simulink model "boostObserver_old"  (R2020a)
settings: Solver=VariableStepAuto  StartTime=0.0  StopTime=3.2  FixedStep=0.0005  MaxStep=9e-06  RelTol=1e-03  EnableMultiTasking=on
InitFcn:
  | kp=0.01;
  | ki=0.01;
  | 
  | k=2;
  | em=100000000;
  | GE=1/em;
  | GU=k*ki/GE;
  | GCE=k*kp/GU;
model workspace (MAT data in the model file):
  time = 0.8
values from neighbouring files (symbols this model uses):
  A1 = obj.boostConverter.A1    [BoostController.m]    (also in BoostConverter.m = [-obj.R/obj.L 0;0 -1/(obj.Ro*obj.C)]; BuckBoostConverter.m = [-obj.R/obj.L 0;0 -1/(obj.Ro*obj.C)]; obsmc.m = Asigma{1,1}; workspace_atual.mat = [-16.4  0; 0  -3.50877192982])
  A2 = obj.boostConverter.A2    [BoostController.m]    (also in BoostConverter.m = [-obj.R/obj.L -1/obj.L;1/obj.C -1/(obj.Ro*obj.C)]; BuckBoostConverter.m = [-obj.R/obj.L 1/obj.L;-1/obj.C -1/(obj.Ro*obj.C)]; obsmc.m = Asigma{1,2}; workspace_atual.mat = [-16.4  -200; 350.877192982  -3.50877192982])
  AlarmDeadTime = 0.50    (= 0.5)    [BoostFaultSimulation.m]    (also in workspace_atual.mat; workspace_certo.mat)
  B1 = obj.boostConverter.B1    [BoostController.m]    (also in BoostConverter.m = [1/obj.L;0]; BuckBoostConverter.m = [1/obj.L;0]; obsmc.m = Bsigma{1,1}; workspace_atual.mat = [200 0])
  boost_parameters = [obj.Ro,obj.R,obj.L,obj.C,obj.u]'    [BoostConverter.m]    (also in BuckBoostConverter.m; boostResults2Latex.m = boost.parameters(); workspace_atual.mat = [100 0.082 0.005 0.00285 190]; workspace_certo.mat = [100 0.082 0.005 0.00285 190])
  C = 1e-3    (= 0.001)    [boostResults2Latex.m]
  CiL = [0 1]    [workspace_atual.mat]    (also in workspace_certo.mat)
  Cmatrix = [1  0; 0  1]    [workspace_atual.mat]    (also in workspace_certo.mat)
  CVc = [1 0]    [workspace_atual.mat]    (also in workspace_certo.mat)
  D1 = [1  0; 0  1]    [workspace_atual.mat]    (also in workspace_certo.mat)
  FaultClass = 0    [BoostFaultSimulation.m]    (also in workspace_atual.mat = 1; workspace_certo.mat = 1)
  iLFaultSwitch = 0    [BoostFaultSimulation.m]    (also in workspace_atual.mat; workspace_certo.mat)
  iLFaultTime = 1.70    (= 1.7)    [BoostFaultSimulation.m]    (also in workspace_atual.mat; workspace_certo.mat)
  iLGainFaultFactor = 15    [BoostFaultSimulation.m]    (also in workspace_atual.mat; workspace_certo.mat)
  iLNoiseFaultSwitch = 0    [BoostFaultSimulation.m]    (also in workspace_atual.mat; workspace_certo.mat)
  iLNoiseTime = 1.70    (= 1.7)    [BoostFaultSimulation.m]    (also in workspace_atual.mat; workspace_certo.mat)
  Jth = 2000    [workspace_atual.mat]    (also in workspace_certo.mat)
  L = 1e-3    (= 0.001)    [boostResults2Latex.m]    (also in obsmc.m = sdpvar(3,1,'full'))
  LoadAddResistor = obj.LoadAddFactor*obj.Ro    [BoostFaultSimulation.m]    (also in workspace_atual.mat = 30; workspace_certo.mat = 30)
  LoadAddSignalSwitch = 1    [BoostFaultSimulation.m]    (also in workspace_atual.mat; workspace_certo.mat)
  LoadAddSwitch = 0    [BoostFaultSimulation.m]    (also in workspace_atual.mat; workspace_certo.mat)
  LoadAddTime = 0.90    (= 0.9)    [BoostFaultSimulation.m]    (also in workspace_atual.mat; workspace_certo.mat)
  LoadRemoveResistor = obj.Ro*(1-obj.LoadRemoveFactor)/(obj.LoadRemoveFactor)    [BoostFaultSimulation.m]    (also in workspace_atual.mat = 233.333333333; workspace_certo.mat = 233.333333333)
  LoadRemoveSignalSwitch = 1    [BoostFaultSimulation.m]    (also in workspace_atual.mat; workspace_certo.mat)
  LoadRemoveSwitch = 0    [BoostFaultSimulation.m]    (also in workspace_atual.mat; workspace_certo.mat)
  LoadRemoveTime = 0.90    (= 0.9)    [BoostFaultSimulation.m]    (also in workspace_atual.mat; workspace_certo.mat)
  LobsiL = [1737913.15707 66180.0912281]    [workspace_atual.mat]    (also in workspace_certo.mat)
  LobsVc = [61200 1]    [workspace_atual.mat]    (also in workspace_certo.mat)
  ObsEp = 70    [workspace_atual.mat]    (also in workspace_certo.mat)
  R = 0.1    [boostResults2Latex.m]    (also in workspace_atual.mat = 0.082; workspace_certo.mat = 0.082)
  ReconfigDelay = 0    [BoostFaultSimulation.m]    (also in workspace_atual.mat = 0.2; workspace_certo.mat = 0.2)
  ReconfigSwitch = 0    [BoostFaultSimulation.m]    (also in workspace_atual.mat; workspace_certo.mat)
  ReconfigTime = 1.707    [BoostFaultSimulation.m]    (also in workspace_atual.mat; workspace_certo.mat)
  rho = 5    [workspace_atual.mat]    (also in workspace_certo.mat)
  RMSfrequency = 47.61    [BoostFaultSimulation.m]    (also in workspace_atual.mat; workspace_certo.mat)
  Ro = 100    [BoostFaultSimulation.m]    (also in boostResults2Latex.m = 10; workspace_atual.mat; workspace_certo.mat)
  Smep = 80    [workspace_atual.mat]    (also in workspace_certo.mat)
  SourceAddSignalSwitch = 1    [BoostFaultSimulation.m]    (also in workspace_atual.mat; workspace_certo.mat)
  SourceAddSwitch = 0    [BoostFaultSimulation.m]    (also in workspace_atual.mat; workspace_certo.mat)
  SourceAddTime = 0.90    (= 0.9)    [BoostFaultSimulation.m]    (also in workspace_atual.mat; workspace_certo.mat)
  SourceAddVoltage = obj.SourceAddFactor*obj.u    [BoostFaultSimulation.m]    (also in workspace_atual.mat = 19; workspace_certo.mat = 19)
  SourceRemoveSignalSwitch = 1    [BoostFaultSimulation.m]    (also in workspace_atual.mat; workspace_certo.mat)
  SourceRemoveSwitch = 0    [BoostFaultSimulation.m]    (also in workspace_atual.mat; workspace_certo.mat)
  SourceRemoveTime = 0.90    (= 0.9)    [BoostFaultSimulation.m]    (also in workspace_atual.mat; workspace_certo.mat)
  SourceRemoveVoltage = obj.SourceRemoveFactor*obj.u    [BoostFaultSimulation.m]    (also in workspace_atual.mat = 19; workspace_certo.mat = 19)
  ueq = 0.5    [workspace_atual.mat]    (also in workspace_certo.mat)
  VcFaultSwitch = 0    [BoostFaultSimulation.m]    (also in workspace_atual.mat; workspace_certo.mat)
  VcFaultTime = 1.70    (= 1.7)    [BoostFaultSimulation.m]    (also in workspace_atual.mat; workspace_certo.mat)
  VcGainFaultFactor = 15    [BoostFaultSimulation.m]    (also in workspace_atual.mat; workspace_certo.mat)
  VcNoiseFaultSwitch = 0    [BoostFaultSimulation.m]    (also in workspace_atual.mat; workspace_certo.mat)
  VcNoiseTime = 1.70    (= 1.7)    [BoostFaultSimulation.m]    (also in workspace_atual.mat; workspace_certo.mat)
  ve = 380    [BoostFaultSimulation.m]    (also in boostResults2Latex.m = 100; workspace_atual.mat; workspace_certo.mat)
  x_e = [ie;ve]    [BoostConverter.m]    (also in BuckBoostConverter.m)
  xe = obj.boostConverter.equilibriumstate(ve)    [BoostController.m]    (also in workspace_atual.mat = [7.62509288104 380]; workspace_certo.mat = [7.62509288104 380])
undefined symbols (not defined in the file or in its folder): Atilde1, Atilde2, Ctilde1, Dtilde1, Dtilde2, F, G, MAXnet, MINnet
libraries: neural x74, powerlib x70, dspstat3 x16, simulink x9, powerlib_meascontrol x7, dspmtrx3 x7, dspmathops x3
(part 7 of 7)

== system boostObserver_old/reset/Fault Identification Neural Netowrk/Pattern Recognition Neural Network3/Layer 2/LW{2,1} ==
  "ad{2,1}" : Inport  PortDimensions=7
      mask Display: e = 0.06;c1 = [120 230 180]/255;c2 = ([120 230 180]+0)/(256+128);c3 = ([120 230 180]+128)/(256+128);patch([0 1 1 0],[0 0 1 1],c1);patch([0 1 1 1-e 1-e 0+e],[0 0 1 1-e 0+e 0+e],c2);patch([0 0 1 1-e 0+e 0+e],[0 1 1 1-e 1-e 0+e],c3);plot([0 1 1 0 0],[0 0 1 1 0]);
  "IW{2,1}(1,:)'" : Constant  Value=[-0.66189722992665156464653364309924654662609100341796875;-0.88643574542094250023893664547358639538288116455078125;2.13457808254518699442314755287952721118927001953125;6.085356418695955227349259075708687305450439453125;21.22403806430467199106715270318090915679931640625;-6.32083600579496529547895988798700273036956787109375;9.282427123435009974627973861061036586761474609375]
      mask Display: e = 0.06;c1 = [120 150 230]/255;c2 = ([120 150 230]+0)/383;c3 = ([120 150 230]+128)/383;patch([0 1 1 0],[0 0 1 1],c1);patch([0 1 1 1-e 1-e 0+e],[0 0 1 1-e 0+e 0+e],c2);patch([0 0 1 1-e 0+e 0+e],[0 1 1 1-e 1-e 0+e],c3);plot([0 1 1 0 0],[0 0 1 1 0]);disp('weights');
  "IW{2,1}(2,:)'" : Constant  Value=[-0.4804089853042199376176313307951204478740692138671875;1.9679320386171015311305154682486318051815032958984375;-2.692357339795323323272668858407996594905853271484375;6.341041197565314035955452709458768367767333984375;-11.476906047142055200538379722274839878082275390625;-2.453294569631040200619054303388111293315887451171875;3.74387294779715507075934510794468224048614501953125]
      mask Display: e = 0.06;c1 = [120 150 230]/255;c2 = ([120 150 230]+0)/383;c3 = ([120 150 230]+128)/383;patch([0 1 1 0],[0 0 1 1],c1);patch([0 1 1 1-e 1-e 0+e],[0 0 1 1-e 0+e 0+e],c2);patch([0 0 1 1-e 0+e 0+e],[0 1 1 1-e 1-e 0+e],c3);plot([0 1 1 0 0],[0 0 1 1 0]);disp('weights');
  "IW{2,1}(3,:)'" : Constant  Value=[5.3247825665589676447098099743016064167022705078125;4.53400579788046531604095434886403381824493408203125;5.8605203546072743847616948187351226806640625;-3.57873441377043643996103128301911056041717529296875;-3.797836814425323392896416407893411815166473388671875;7.5391462496435348583645463804714381694793701171875;-16.35436033871092575964212301187217235565185546875]
      mask Display: e = 0.06;c1 = [120 150 230]/255;c2 = ([120 150 230]+0)/383;c3 = ([120 150 230]+128)/383;patch([0 1 1 0],[0 0 1 1],c1);patch([0 1 1 1-e 1-e 0+e],[0 0 1 1-e 0+e 0+e],c2);patch([0 0 1 1-e 0+e 0+e],[0 1 1 1-e 1-e 0+e],c3);plot([0 1 1 0 0],[0 0 1 1 0]);disp('weights');
  "IW{2,1}(4,:)'" : Constant  Value=[-0.044411847017804373383143001774442382156848907470703125;0.24171277236156896162100338187883608043193817138671875;2.848562710208792925214993374538607895374298095703125;-15.870262410075898884542766609229147434234619140625;4.62155800806790839629911715746857225894927978515625;9.4424049491628476715732176671735942363739013671875;-0.78821586059881931785042752380832098424434661865234375]
      mask Display: e = 0.06;c1 = [120 150 230]/255;c2 = ([120 150 230]+0)/383;c3 = ([120 150 230]+128)/383;patch([0 1 1 0],[0 0 1 1],c1);patch([0 1 1 1-e 1-e 0+e],[0 0 1 1-e 0+e 0+e],c2);patch([0 0 1 1-e 0+e 0+e],[0 1 1 1-e 1-e 0+e],c3);plot([0 1 1 0 0],[0 0 1 1 0]);disp('weights');
  "IW{2,1}(5,:)'" : Constant  Value=[-2.263023379485125108345755506888963282108306884765625;-5.144949209871551687456303625367581844329833984375;-7.2575383360688707767849336960352957248687744140625;6.99592241235283740508066330221481621265411376953125;-9.36041695900031101018612389452755451202392578125;-7.83937220230751474758790209307335317134857177734375;5.63846069928163284856736936490051448345184326171875]
      mask Display: e = 0.06;c1 = [120 150 230]/255;c2 = ([120 150 230]+0)/383;c3 = ([120 150 230]+128)/383;patch([0 1 1 0],[0 0 1 1],c1);patch([0 1 1 1-e 1-e 0+e],[0 0 1 1-e 0+e 0+e],c2);patch([0 0 1 1-e 0+e 0+e],[0 1 1 1-e 1-e 0+e],c3);plot([0 1 1 0 0],[0 0 1 1 0]);disp('weights');
  Mux : Mux  Inputs=5
      mask Display: e = 0.06;c1 = [120 150 230]/255;c2 = ([120 150 230]+0)/383;c3 = ([120 150 230]+128)/383;patch([0 1 1 0],[0 0 1 1],c1);patch([0 1 1 1-e 1-e 0+e],[0 0 1 1-e 0+e 0+e],c2);patch([0 0 1 1-e 0+e 0+e],[0 1 1 1-e 1-e 0+e],c3);plot([0 1 1 0 0],[0 0 1 1 0]);disp('Mux');
  dotprod{1..5} (5 alike) : neural/Weight Functions/dotprod
  "lz{2,1}" : Outport
      mask Display: e = 0.06;c1 = [120 230 180]/255;c2 = ([120 230 180]+0)/(256+128);c3 = ([120 230 180]+128)/(256+128);patch([0 1 1 0],[0 0 1 1],c1);patch([0 1 1 1-e 1-e 0+e],[0 0 1 1-e 0+e 0+e],c2);patch([0 0 1 1-e 0+e 0+e],[0 1 1 1-e 1-e 0+e],c3);plot([0 1 1 0 0],[0 0 1 1 0]);
  wires:
  "IW{2,1}(1,:)'"/1 -> dotprod1/1
  "ad{2,1}"/1 -> dotprod1/2, dotprod2/2, dotprod3/2, dotprod4/2, dotprod5/2
  dotprod1/1 -> Mux/1
  "IW{2,1}(2,:)'"/1 -> dotprod2/1
  dotprod2/1 -> Mux/2
  "IW{2,1}(3,:)'"/1 -> dotprod3/1
  dotprod3/1 -> Mux/3
  "IW{2,1}(4,:)'"/1 -> dotprod4/1
  dotprod4/1 -> Mux/4
  "IW{2,1}(5,:)'"/1 -> dotprod5/1
  dotprod5/1 -> Mux/5
  Mux/1 -> "lz{2,1}"/1

== matlab function boostObserver_old/reset/Controlador1/xe ==
  data: boost_parameters input; ve input; x_e output; i_e output
function [x_e,i_e] = fcn(boost_parameters,ve)
%parameters = (Ro,R,L,C,u)
%     
R = boost_parameters(2);
Ro = boost_parameters(1);
u = boost_parameters(5);

delta_ie = (-u/R)^2 - (4*ve^2)/(R*Ro);
i_e = real(((u/R) - sqrt(complex(delta_ie)))/2);  
x_e = [i_e;ve];

== matlab function boostObserver_old/Subsystem3/Controlador1/xe ==
  data: boost_parameters input; ve input; x_e output; i_e output
function [x_e,i_e] = fcn(boost_parameters,ve)
%parameters = (Ro,R,L,C,u)
%     
R = boost_parameters(2);
Ro = boost_parameters(1);
u = boost_parameters(5);

delta_ie = (-u/R)^2 - (4*ve^2)/(R*Ro);
i_e = real(((u/R) - sqrt(complex(delta_ie)))/2);  
x_e = [i_e;ve];

== matlab function boostObserver_old/Subsystem/Controlador1/xe ==
  data: boost_parameters input; ve input; x_e output; i_e output
function [x_e,i_e] = fcn(boost_parameters,ve)
%parameters = (Ro,R,L,C,u)
%     
R = boost_parameters(2);
Ro = boost_parameters(1);
u = boost_parameters(5);

delta_ie = (-u/R)^2 - (4*ve^2)/(R*Ro);
i_e = real(((u/R) - sqrt(complex(delta_ie)))/2);  
x_e = [i_e;ve];
